simulink model "Node_M_3D"  (R2024b)
settings: Solver=ode1  StartTime=0.0  StopTime=10.0  FixedStep=0.5e-3  RelTol=1e-3
model workspace (MAT data in the model file):
  cfg.ax0 = -8.7
  cfg.ay0 = -190.9
  cfg.az0 = -190.4
  cfg.ax1 = -23.6
  cfg.ay1 = -45.5
  cfg.az1 = -12.9
  cfg.ax2 = -6.9
  cfg.ay2 = 75.9
  cfg.az2 = 6826.5
  cfg.ax3 = -17.809705
  cfg.ay3 = 13.971374
  cfg.az3 = 1.783211
  cfg.bx1 = 777.2
  cfg.by1 = 58.9
  cfg.bz1 = 276.6
  cfg.VR = 30
  cfg.VT = 44.5
  cfg.VO = 122.870185
  cfg.a = 0.29
  cfg.b = 62.89
  cfg.c = 0.7
  cfg.d = 10.99
  cfg.e = 0.04
settings Model: DataDictionary=M_dd.sldd  EnableAccessToBaseWorkspace=off  Creator=wai484  LastModifiedBy=wai484
settings SolverCC: EnableFixedStepZeroCrossing=on
settings OptimizationCC: UseDivisionForNetSlopeComputation=UseDivisionForReciprocalsOfIntegersOnly

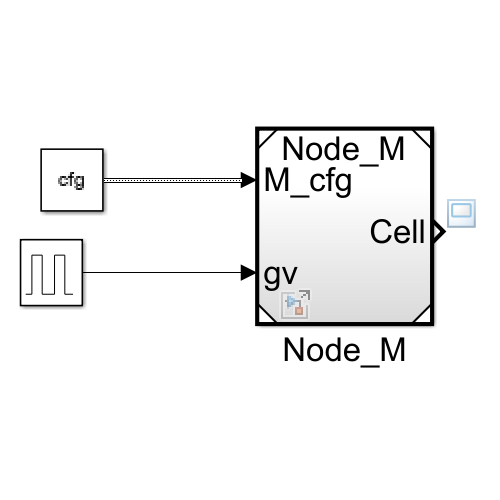
[thumbnail: Simulink's stored preview of the top-level diagram]
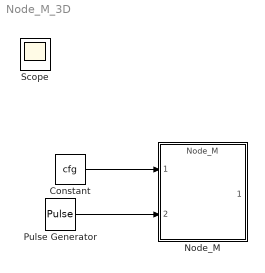
== system Node_M_3D ==
  Constant : Constant  Value=cfg  OutDataTypeStr=Bus: Config_M  SampleTime=-1
  Node_M : ModelReference  ModelNameDialog=Node_M  SimulationMode=Normal  ModelReferenceVersion=1.87
  Pulse Generator : DiscretePulseGenerator  PulseType=Time based  Amplitude=50  Period=1  PulseWidth=5
  Scope : Scope
  wires:
  Constant/1 -> Node_M/1
  Pulse Generator/1 -> Node_M/2
